simulink model "DSMC_params"  (R2020a)
settings: Solver=FixedStepAuto  StartTime=0.0  StopTime=30  FixedStep=Ts  MaxStep=0.015  RelTol=1e-3
PreLoadFcn:
  | if ~exist('sim_HIL')
  |     sim_HIL=false;
  | end
  | if ~exist('usefilter')
  |     usefilter=false;
  | end
InitFcn:
  | load motorModel.mat
  | load expsetup
model workspace (MAT data in the model file):
  C = [50; 1]
  DSMC_params_sdosession = sldodialogs.data.SessionData
  DSMC_params_sdosession.Version = '3.0'
  DSMC_params_sdosession.Data.ModelName = 'DSMC_params'
  DSMC_params_sdosession.Data.ToolType = 'ResponseOptimization'
  DSMC_params_sdosession.Data.GUIOptions.NoPromptClose = 0
  DSMC_params_sdosession.Data.Workspace.LocalWorkspace.DesignVars(1) = param.Continuous
  DSMC_params_sdosession.Data.Workspace.LocalWorkspace.DesignVars(1).Scale_ = [4; 1]
  DSMC_params_sdosession.Data.Workspace.LocalWorkspace.DesignVars(1).Size_ = [2 1]
  DSMC_params_sdosession.Data.Workspace.LocalWorkspace.DesignVars(1).Value_ = [50; 1]
  DSMC_params_sdosession.Data.Workspace.LocalWorkspace.DesignVars(1).pID = paramid.Variable
  DSMC_params_sdosession.Data.Workspace.LocalWorkspace.DesignVars(1).pID.Name = 'C'
  DSMC_params_sdosession.Data.Workspace.LocalWorkspace.DesignVars(2) = param.Continuous
  DSMC_params_sdosession.Data.Workspace.LocalWorkspace.DesignVars(2).Minimum_ = 1e-05
  DSMC_params_sdosession.Data.Workspace.LocalWorkspace.DesignVars(2).Maximum_ = 0.99999
  DSMC_params_sdosession.Data.Workspace.LocalWorkspace.DesignVars(2).Scale_ = 0.25
  DSMC_params_sdosession.Data.Workspace.LocalWorkspace.DesignVars(2).Size_ = [1 1]
  DSMC_params_sdosession.Data.Workspace.LocalWorkspace.DesignVars(2).Value_ = 0.1
  DSMC_params_sdosession.Data.Workspace.LocalWorkspace.DesignVars(2).pID = paramid.Variable
  DSMC_params_sdosession.Data.Workspace.LocalWorkspace.DesignVars(2).pID.Name = 'del'
  DSMC_params_sdosession.Data.Workspace.LocalWorkspace.DesignVars(3) = param.Continuous
  DSMC_params_sdosession.Data.Workspace.LocalWorkspace.DesignVars(3).Minimum_ = 1e-05
  DSMC_params_sdosession.Data.Workspace.LocalWorkspace.DesignVars(3).Maximum_ = 50
  DSMC_params_sdosession.Data.Workspace.LocalWorkspace.DesignVars(3).Scale_ = 0.001
  DSMC_params_sdosession.Data.Workspace.LocalWorkspace.DesignVars(3).Size_ = [1 1]
  DSMC_params_sdosession.Data.Workspace.LocalWorkspace.DesignVars(3).Value_ = 1
  DSMC_params_sdosession.Data.Workspace.LocalWorkspace.DesignVars(3).pID = paramid.Variable
  DSMC_params_sdosession.Data.Workspace.LocalWorkspace.DesignVars(3).pID.Name = 'eta'
  DSMC_params_sdosession.Data.Workspace.LocalWorkspace.DesignVars(4) = param.Continuous
  DSMC_params_sdosession.Data.Workspace.LocalWorkspace.DesignVars(4).Minimum_ = 1
  DSMC_params_sdosession.Data.Workspace.LocalWorkspace.DesignVars(4).Maximum_ = 100
  DSMC_params_sdosession.Data.Workspace.LocalWorkspace.DesignVars(4).Size_ = [1 1]
  DSMC_params_sdosession.Data.Workspace.LocalWorkspace.DesignVars(4).Value_ = 20
  DSMC_params_sdosession.Data.Workspace.LocalWorkspace.DesignVars(4).pID = paramid.Variable
  DSMC_params_sdosession.Data.Workspace.LocalWorkspace.DesignVars(4).pID.Name = 'gamm'
  DSMC_params_sdosession.Data.Workspace.LocalWorkspace.DesignVars(5) = param.Continuous
  DSMC_params_sdosession.Data.Workspace.LocalWorkspace.DesignVars(5).Minimum_ = 1e-05
  DSMC_params_sdosession.Data.Workspace.LocalWorkspace.DesignVars(5).Maximum_ = 0.99999
  DSMC_params_sdosession.Data.Workspace.LocalWorkspace.DesignVars(5).Scale_ = 0.5
  DSMC_params_sdosession.Data.Workspace.LocalWorkspace.DesignVars(5).Size_ = [1 1]
  DSMC_params_sdosession.Data.Workspace.LocalWorkspace.DesignVars(5).Value_ = 0.1
  DSMC_params_sdosession.Data.Workspace.LocalWorkspace.DesignVars(5).pID = paramid.Variable
  DSMC_params_sdosession.Data.Workspace.LocalWorkspace.DesignVars(5).pID.Name = 'qT'
  DSMC_params_sdosession.Data.Workspace.LocalWorkspace.DesignVars(6) = param.Continuous
  DSMC_params_sdosession.Data.Workspace.LocalWorkspace.DesignVars(6).Minimum_ = 1e-05
  DSMC_params_sdosession.Data.Workspace.LocalWorkspace.DesignVars(6).Maximum_ = 50
  DSMC_params_sdosession.Data.Workspace.LocalWorkspace.DesignVars(6).Scale_ = 0.5
  DSMC_params_sdosession.Data.Workspace.LocalWorkspace.DesignVars(6).Size_ = [1 1]
  DSMC_params_sdosession.Data.Workspace.LocalWorkspace.DesignVars(6).Value_ = 1
  DSMC_params_sdosession.Data.Workspace.LocalWorkspace.DesignVars(6).pID = paramid.Variable
  DSMC_params_sdosession.Data.Workspace.LocalWorkspace.DesignVars(6).pID.Name = 'vphi'
  DSMC_params_sdosession.Data.Workspace.LocalWorkspace.DesignVars(7) = param.Continuous
  DSMC_params_sdosession.Data.Workspace.LocalWorkspace.DesignVars(7).Minimum_ = 1e-05
  DSMC_params_sdosession.Data.Workspace.LocalWorkspace.DesignVars(7).Maximum_ = 50
  DSMC_params_sdosession.Data.Workspace.LocalWorkspace.DesignVars(7).Scale_ = 0.5
  DSMC_params_sdosession.Data.Workspace.LocalWorkspace.DesignVars(7).Size_ = [1 1]
  DSMC_params_sdosession.Data.Workspace.LocalWorkspace.DesignVars(7).Value_ = 10
  DSMC_params_sdosession.Data.Workspace.LocalWorkspace.DesignVars(7).pID = paramid.Variable
  DSMC_params_sdosession.Data.Workspace.LocalWorkspace.DesignVars(7).pID.Name = 'xiT'
  DSMC_params_sdosession.Data.Workspace.LocalWorkspace.posErr = Simulink.SimulationData.Signal
  DSMC_params_sdosession.Data.Workspace.LocalWorkspace.posErr.PortType = 'outport'
  DSMC_params_sdosession.Data.Workspace.LocalWorkspace.posErr.Version = 1
  DSMC_params_sdosession.Data.Workspace.LocalWorkspace.posErr.BlockPath = Simulink.SimulationData.BlockPath
  DSMC_params_sdosession.Data.Workspace.LocalWorkspace.posErr.BlockPath.path = {'DSMC_params/Visualization/Minus'}
  DSMC_params_sdosession.Data.Workspace.LocalWorkspace.posErrTracking = sdo.requirements.SignalTracking
  DSMC_params_sdosession.Data.Workspace.LocalWorkspace.posErrTracking.any.ReferenceSignal = timeseries
  DSMC_params_sdosession.Data.Workspace.LocalWorkspace.posErrTracking.any.ReferenceSignal.Name = 'unnamed'
  DSMC_params_sdosession.Data.Workspace.LocalWorkspace.posErrTracking.any.ReferenceSignal.DataInfo = tsdata.datametadata
  DSMC_params_sdosession.Data.Workspace.LocalWorkspace.posErrTracking.any.ReferenceSignal.DataInfo.Interpolation = tsdata.interpolation
  DSMC_params_sdosession.Data.Workspace.LocalWorkspace.posErrTracking.any.ReferenceSignal.DataInfo.Interpolation.Fhandle : function handle (value not decoded)
  DSMC_params_sdosession.Data.Workspace.LocalWorkspace.posErrTracking.any.ReferenceSignal.DataInfo.Interpolation.Name = 'linear'
  DSMC_params_sdosession.Data.Workspace.LocalWorkspace.posErrTracking.any.ReferenceSignal.TimeInfo = tsdata.timemetadata
  DSMC_params_sdosession.Data.Workspace.LocalWorkspace.posErrTracking.any.ReferenceSignal.TimeInfo.Length = 2
  DSMC_params_sdosession.Data.Workspace.LocalWorkspace.posErrTracking.any.ReferenceSignal.TimeInfo.DuplicateTimes = 0
  DSMC_params_sdosession.Data.Workspace.LocalWorkspace.posErrTracking.any.ReferenceSignal.TimeInfo.Time_ = [0; 30]
  DSMC_params_sdosession.Data.Workspace.LocalWorkspace.posErrTracking.any.ReferenceSignal.TimeInfo.Initialized = 1
  DSMC_params_sdosession.Data.Workspace.LocalWorkspace.posErrTracking.any.ReferenceSignal.QualityInfo = tsdata.qualmetadata
  DSMC_params_sdosession.Data.Workspace.LocalWorkspace.posErrTracking.any.ReferenceSignal.Data_ = [0; 0]
  DSMC_params_sdosession.Data.Workspace.LocalWorkspace.posErrTracking.any.Weights = [1; 1]
  DSMC_params_sdosession.Data.Workspace.LocalWorkspace.posErrTracking.any.Type = '=='
  DSMC_params_sdosession.Data.Workspace.LocalWorkspace.posErrTracking.any.Method = 'SSE'
  DSMC_params_sdosession.Data.Workspace.LocalWorkspace.posErrTracking.any.InterpolationTimes = 'Reference only'
  DSMC_params_sdosession.Data.Workspace.LocalWorkspace.posErrTracking.any.Normalize = 'on'
  DSMC_params_sdosession.Data.Workspace.LocalWorkspace.posErrTracking.any.RobustCost = 'on'
  DSMC_params_sdosession.Data.Workspace.LocalWorkspace.posErrTracking.any.RelTol = 0
  DSMC_params_sdosession.Data.Workspace.LocalWorkspace.posErrTracking.any.AbsTol = 0
  DSMC_params_sdosession.Data.Workspace.LocalWorkspace.posErrTracking.any.Name = ''
  DSMC_params_sdosession.Data.Workspace.LocalWorkspace.posErrTracking.any.Description = ''
  DSMC_params_sdosession.Data.Workspace.LocalWorkspace.posLowerBound = sdo.requirements.SignalBound
  DSMC_params_sdosession.Data.Workspace.LocalWorkspace.posLowerBound.sdo.requirements.Requirement.Data_ : srorequirement.piecewisedata (value not decoded)
  DSMC_params_sdosession.Data.Workspace.LocalWorkspace.posLowerBound.sdo.requirements.Requirement.Check_ = sdo.requirements.PiecewiseLinearCheck
  DSMC_params_sdosession.Data.Workspace.LocalWorkspace.posLowerBound.sdo.requirements.Requirement.Check_.Orientation = 'horizontal'
  DSMC_params_sdosession.Data.Workspace.LocalWorkspace.posLowerBound.sdo.requirements.Requirement.Check_.XScale = 'linear'
  DSMC_params_sdosession.Data.Workspace.LocalWorkspace.posUpperBound = sdo.requirements.SignalBound
  DSMC_params_sdosession.Data.Workspace.LocalWorkspace.posUpperBound.sdo.requirements.Requirement.Data_ : srorequirement.piecewisedata (value not decoded)
  DSMC_params_sdosession.Data.Workspace.LocalWorkspace.posUpperBound.sdo.requirements.Requirement.Check_ = sdo.requirements.PiecewiseLinearCheck
  DSMC_params_sdosession.Data.Workspace.LocalWorkspace.posUpperBound.sdo.requirements.Requirement.Check_.Orientation = 'horizontal'
  DSMC_params_sdosession.Data.Workspace.LocalWorkspace.posUpperBound.sdo.requirements.Requirement.Check_.XScale = 'linear'
  DSMC_params_sdosession.Data.Workspace.LocalWorkspace.velErr = Simulink.SimulationData.Signal
  DSMC_params_sdosession.Data.Workspace.LocalWorkspace.velErr.PortType = 'outport'
  DSMC_params_sdosession.Data.Workspace.LocalWorkspace.velErr.Version = 1
  DSMC_params_sdosession.Data.Workspace.LocalWorkspace.velErr.BlockPath = Simulink.SimulationData.BlockPath
  DSMC_params_sdosession.Data.Workspace.LocalWorkspace.velErr.BlockPath.path = {'DSMC_params/Visualization/Minus4'}
  DSMC_params_sdosession.Data.Workspace.HiddenWorkspace = []
  DSMC_params_sdosession.Data.ToolData.PlotManager.Plots.Class = 'sldoplots.TimePlot'
  DSMC_params_sdosession.Data.ToolData.PlotManager.Plots.Sources = {'posErr'}
  DSMC_params_sdosession.Data.ToolData.PlotManager.Tiling : java.lang.String (value not decoded)
  DSMC_params_sdosession.Data.ToolData.DialogManager = []
  DSMC_params_sdosession.Data.ToolData.ResponseOptimization.Options = sdo.OptimizeOptions
  DSMC_params_sdosession.Data.ToolData.ResponseOptimization.Options.OptimizedModel = 'SMC2'
  DSMC_params_sdosession.Data.ToolData.ResponseOptimization.Options.Version = 2
  DSMC_params_sdosession.Data.ToolData.ResponseOptimization.GUIOptions.ModelTimeOut = Inf
  DSMC_params_sdosession.Data.ToolData.ResponseOptimization.GUIOptions.ComputeOperatingPoint = 0
  DSMC_params_sdosession.Data.ToolData.ResponseOptimization.GUIOptions.ShowProgress = 1
  DSMC_params_sdosession.Data.ToolData.ResponseOptimization.GUIOptions.ShowParamTrajectory = 1
  DSMC_params_sdosession.Data.ToolData.ResponseOptimization.GUIOptions.UpdatePlots = 1
  DSMC_params_sdosession.Data.ToolData.ResponseOptimization.GUIOptions.UpdateModel = 1
  DSMC_params_sdosession.Data.ToolData.ResponseOptimization.GUIOptions.UpdateDesign = 'overwrite'
  DSMC_params_sdosession.Data.ToolData.ResponseOptimization.GUIOptions.SaveReport = 0
  DSMC_params_sdosession.Data.ToolData.ResponseOptimization.GUIOptions.SaveRequirementValue = 1
  DSMC_params_sdosession.Data.ToolData.ResponseOptimization.LinOptions = linearize.LinearizeOptions
  DSMC_params_sdosession.Data.ToolData.ResponseOptimization.RequirementOperatingPointSetup = []
  DSMC_params_sdosession.Data.ToolData.ResponseOptimization.LocalRequirements(1).Requirement = 'posErrTracking'
  DSMC_params_sdosession.Data.ToolData.ResponseOptimization.LocalRequirements(1).Source = {'posErr'}
  DSMC_params_sdosession.Data.ToolData.ResponseOptimization.LocalRequirements(1).Selected = 1
  DSMC_params_sdosession.Data.ToolData.ResponseOptimization.LocalRequirements(2).Requirement = 'posUpperBound'
  DSMC_params_sdosession.Data.ToolData.ResponseOptimization.LocalRequirements(2).Source = {'posErr'}
  DSMC_params_sdosession.Data.ToolData.ResponseOptimization.LocalRequirements(2).Selected = 1
  DSMC_params_sdosession.Data.ToolData.ResponseOptimization.LocalRequirements(3).Requirement = 'posLowerBound'
  DSMC_params_sdosession.Data.ToolData.ResponseOptimization.LocalRequirements(3).Source = {'posErr'}
  DSMC_params_sdosession.Data.ToolData.ResponseOptimization.LocalRequirements(3).Selected = 1
  DSMC_params_sdosession.Data.ToolData.ResponseOptimization.BlockRequirements = struct([])
  DSMC_params_sdosession.Data.ToolData.ResponseOptimization.LocalExperiments = struct([])
  DSMC_params_sdosession.Data.ToolData.ResponseOptimization.Cost.Type = 'SSE'
  DSMC_params_sdosession.Data.ToolData.ResponseOptimization.Cost.Robust = 'off'
  DSMC_params_sdosession.Data.ToolData.ResponseOptimization.DesignVariables = 'DesignVars'
  DSMC_params_sdosession.Data.ToolData.ResponseOptimization.UncertainVariables = ''
  DSMC_params_sdosession.Data.ToolData.ResponseOptimization.DataToPlot = 'posLowerBound'
  N = 10
  Ts_path = 0.015
  del = 0.1
  eta = 1
  gamm = 20
  nodeID = 4
  qT = 0.1
  vphi = 1
  xiT = 10
values from neighbouring files (symbols this model uses):
  Ts = 0.02    [PolynomialFit.m]
undefined symbols (not defined in the file or in its folder): k_lp, mModel, tau_lp, x28_000006_reduction
undefined symbols (not defined in the file): k, Xd
libraries: eeGeneralControl x1, dspsrcs4 x1, simulink_extras x1, simulink x1
settings Model: DataDictionary=MotorInfo.sldd  SimulationMode=accelerator  OrderedModelArguments=off  Creator=khoi  LastModifiedBy=khoi
settings OptimizationCC: DefaultParameterBehavior=Inlined  UseDivisionForNetSlopeComputation=on  GainParamInheritBuiltInType=on  UseFloatMulNetSlope=on  InlineInvariantSignals=on  EnhancedBackFolding=on  PassReuseOutputArgsAs=Individual arguments  ZeroExternalMemoryAtStartup=off  ZeroInternalMemoryAtStartup=off  EfficientFloat2IntCast=on  LifeSpan=50  SimCompilerOptimization=on  OptimizeBlockOrder=speed  DifferentSizesBufferReuse=on  OptimizationCustomize=off  EfficientTunableParamExpr=on
settings DebuggingCC: SignalInfNanChecking=warning  ParameterTunabilityLossMsg=error  AssertControl=DisableAll  SFUndirectedBroadcastEventsDiag=error
settings HardwareCC: ProdLongLongMode=on
settings ModelReferenceCC: EnableRefExpFcnMdlSchedulingChecks=off  EnableParallelModelReferenceBuilds=on  ModelReferenceMinAlgLoopOccurrences=on
settings SFSimCC: SimParseCustomCode=off  CompileTimeRecursionLimit=0  EnableRuntimeRecursion=off  MATLABDynamicMemAlloc=off
settings RTWCC: SystemTargetFile=ert.tlc  GenCodeOnly=on  TemplateMakefile=ert_default_tmf  GenerateReport=on  LaunchReport=on  CheckMdlBeforeBuild=Warning
settings CodeAppCC: ForceParamTrailComments=on  IgnoreCustomStorageClasses=off  OperatorAnnotations=on  SimulinkDataObjDesc=on  SFDataObjDesc=on  MATLABFcnDesc=on  InsertBlockDesc=on
settings ERTTargetCC: TargetLangStandard=C99 (ISO)  UtilityFuncGeneration=Shared location  GenerateSampleERTMain=on  SupportNonFinite=off  ParenthesesLevel=Maximum  CastingMode=Standards  GenerateSharedConstants=off  InlinedParameterPlacement=NonHierarchical  ERTCustomFileTemplate=example_file_process.tlc  EnableSignedLeftShifts=off  EnableSignedRightShifts=off

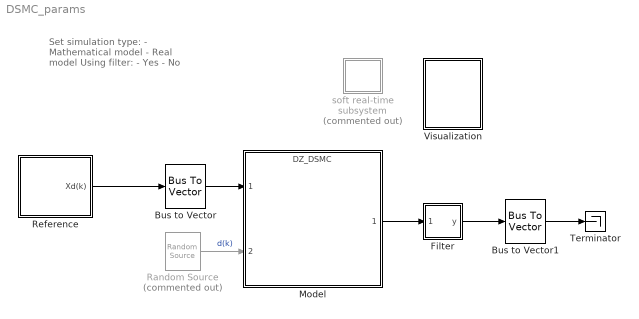
== system DSMC_params ==
  note: Set simulation type:
      | - Mathematical model
      | - Real model
      | Using filter:
      | - Yes
      | - No
  Bus to Vector : BusToVector
  Bus to Vector1 : BusToVector
  Filter : Subsystem
  Model : ModelReference  ModelNameDialog=DZ_DSMC.slx  ModelReferenceVersion=1.699  mask{Phi=mModel{nodeID,3}.A, Gam=mModel{nodeID,3}.B, nodeID=0, C=C, qT=qT, xiT=xiT, delt=del, vphi=vphi, eta=eta, gamm=gamm, Ts=Ts, N=N}
      mask prompts: Phi "State matrix"; Gam "Input matrix"; nodeID "Node ID"; C "Sliding vector"; qT "qT (0<1-qT<1)"; xiT "xiT >0"; delt "0<delta<1"; vphi "vphi>0"; eta "eta >0"; gamm "gamma (positive natural number)"; Ts "Sample tiem"; N "N order"
  Random Source : dspsrcs4/Random Source  Commented=on  SrcType=Gaussian  NormMethod=Ziggurat  CltLength=12  MinVal=0  MaxVal=1  MeanVal=0  VarVal=1  RepMode=Not repeatable  rawSeed=1  IsInherit=off  SampMode=Discrete  SampTime=Ts  SampFrame=1  DataType=Double  OutComplex=Real  OutputFrames=off
  Reference : Subsystem
  Terminator : Terminator
  Visualization : Subsystem
  soft real-time subsystem : Subsystem  Commented=on  mask{t_sample=0.01}
      mask prompts: t_sample "Sleep function interval (s)"
  wires:
  Reference/1(Xd(k)) -> Bus to Vector/1
  Filter/1(y) -> Bus to Vector1/1
  Random Source/1 -> Model/2  "d(k)"
  Bus to Vector/1 -> Model/1
  Bus to Vector1/1 -> Terminator/1
  Model/1 -> Filter/1(Input)

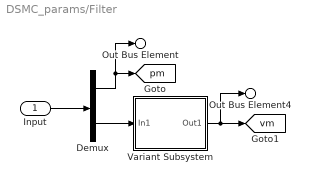
== system DSMC_params/Filter ==
  Input : Inport
  Demux : Demux  Outputs=2
  Variant Subsystem : Subsystem  Variant=on
  Out Bus Element4 : Outport  PortName=y  Element=dx
  Out Bus Element : Outport  PortName=y  Element=x
  tag scope: pm=global, vm=global
  wires:
  Demux/2 -> Variant Subsystem/1(In1)
  Demux/1 -> [pm], Out Bus Element/1
  Variant Subsystem/1(Out1) -> [vm], Out Bus Element4/1
  Input/1 -> Demux/1

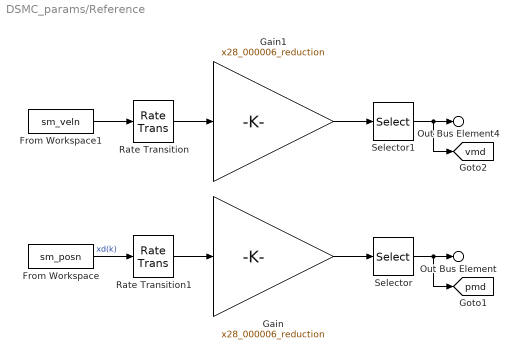
== system DSMC_params/Reference ==
  From Workspace : FromWorkspace  VariableName=sm_posn  SampleTime=Ts_path
  From Workspace1 : FromWorkspace  VariableName=sm_veln  SampleTime=Ts_path
  Gain : Gain  Gain=x28_000006_reduction
  Gain1 : Gain  Gain=x28_000006_reduction
  Rate Transition : RateTransition  OutPortSampleTime=Ts
  Rate Transition1 : RateTransition  OutPortSampleTime=Ts
  Selector : Selector  InputPortWidth=4  IndexOptions=Index vector (dialog)  Indices=nodeID  OutputSizes=1
  Selector1 : Selector  InputPortWidth=4  IndexOptions=Index vector (dialog)  Indices=nodeID  OutputSizes=1
  Out Bus Element : Outport  PortName=Xd(k)  Element=m.x
  Out Bus Element4 : Outport  PortName=Xd(k)  Element=m.dx
  tag scope: pmd=global, vmd=global
  wires:
  Selector1/1 -> [vmd], Out Bus Element4/1
  Selector/1 -> [pmd], Out Bus Element/1
  Gain/1 -> Selector/1
  From Workspace/1 -> Rate Transition1/1  "xd(k)"
  From Workspace1/1 -> Rate Transition/1
  Gain1/1 -> Selector1/1
  Rate Transition/1 -> Gain1/1
  Rate Transition1/1 -> Gain/1

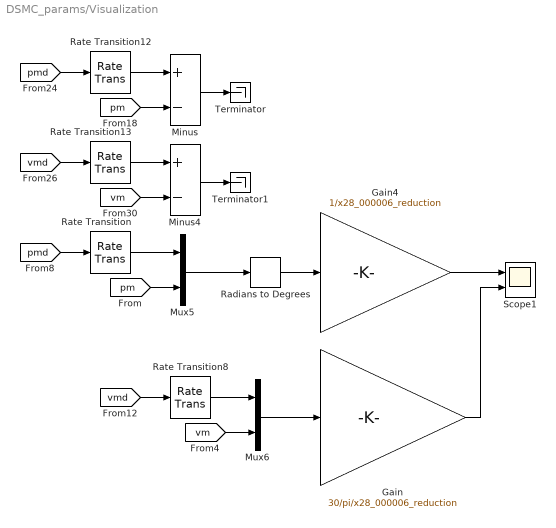
== system DSMC_params/Visualization ==
  Gain : Gain  Gain=30/pi/x28_000006_reduction
  Gain4 : Gain  Gain=1/x28_000006_reduction
  Minus : Sum  Inputs=+-
  Minus4 : Sum  Inputs=+-
  Mux5 : Mux  Inputs=2
  Mux6 : Mux  Inputs=2
  Radians to Degrees : simulink_extras/Transformations/Radians to Degrees
  Rate Transition{,8,12..13} (4 alike) : RateTransition
  Scope1 : Scope  NumInputPorts=2
  Terminator : Terminator
  Terminator1 : Terminator
  wires:
  Rate Transition8/1 -> Mux6/1
  Rate Transition13/1 -> Minus4/1
  Radians to Degrees/1 -> Gain4/1
  Rate Transition12/1 -> Minus/1
  [pm] -> Minus/2
  [vmd] -> Rate Transition13/1
  [vmd] -> Rate Transition8/1
  Gain4/1 -> Scope1/1
  Rate Transition/1 -> Mux5/1
  [vm] -> Minus4/2
  [pmd] -> Rate Transition12/1
  [vm] -> Mux6/2
  [pm] -> Mux5/2
  Mux5/1 -> Radians to Degrees/1
  [pmd] -> Rate Transition/1
  Minus/1 -> Terminator/1
  Mux6/1 -> Gain/1
  Gain/1 -> Scope1/2
  Minus4/1 -> Terminator1/1

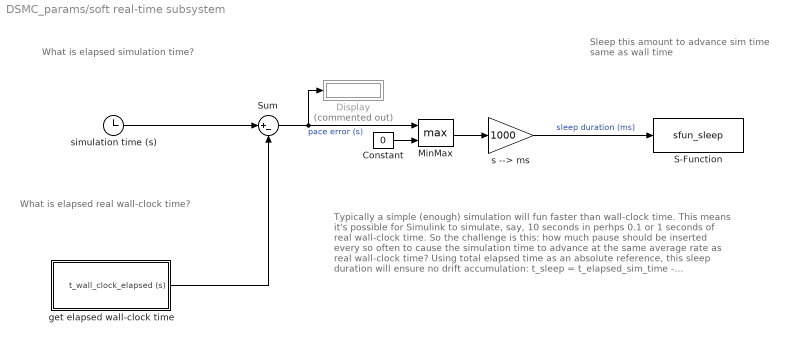
== system DSMC_params/soft real-time subsystem ==
  note: What is elapsed real
      | wall-clock time?
  note: What is elapsed
      | simulation time?
  note: Sleep this amount
      | to advance sim time
      | same as wall time
  note: Typically a simple (enough) simulation will fun faster than
      | wall-clock time. This means it's possible for Simulink to
      | simulate, say, 10 seconds in perhps 0.1 or 1 seconds of real
      | wall-clock time.
      |
      | So the challenge is this: how much pause should be inserted
      | every so often to cause the simulation time to advance at
      | the same average rate as real wall-clock time?
      |
      | Using total elapsed time as an absolute reference, this
      | sleep duration will ensure no drift accumulation:
      |
      | t_sleep = t_elapsed_sim_time - t_elapsed_wall_clock_time
      |
      | Pace error and Sleep() or usleep() resolution is system dependent
      | and likely around 10ms on Windows machines. Better on linux.
      |
      | Marc Compere
      | comperem@gmail.com
      | created : 28 May 2018
      | modified: 29 May 2018
      |
      | Reference:
      | Marc Compere (2022). S oft Real Time Block for Pacing Simulink Simulations (https://www.mathworks.com/matlabcentral/fileexchange/67520-soft-real-time-block-for-pacing-simulink-simulations), MATLAB Central File Exchange. Retrieved March 14, 2022.
  Constant : Constant  Value=0
  Display : Display  Commented=on
  MinMax : MinMax  Function=max  Inputs=2
  S-Function : S-Function  FunctionName=sfun_sleep  Parameters=t_sample  SFunctionDeploymentMode=off  EnableBusSupport=off
  Sum : Sum  Inputs=|+-
  get elapsed wall-clock time : Subsystem
  s --> ms : Gain  Gain=1000
  simulation time (s) : Clock
  wires:
  simulation time (s)/1 -> Sum/1
  Constant/1 -> MinMax/2
  get elapsed wall-clock time/1(t_wall_clock_elapsed (s)) -> Sum/2
  Sum/1 -> Display/1, MinMax/1  "pace error (s)"
  MinMax/1 -> s --> ms/1
  s --> ms/1 -> S-Function/1  "sleep duration (ms)"

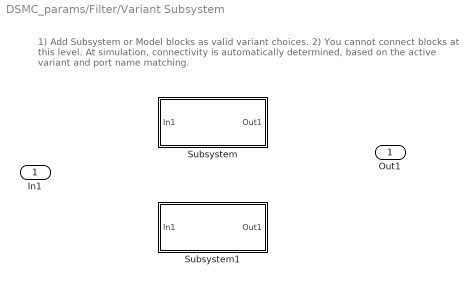
== system DSMC_params/Filter/Variant Subsystem ==
  note: 1) Add Subsystem or Model blocks as valid variant choices.
      | 2) You cannot connect blocks at this level. At simulation, connectivity is automatically
      | determined, based on the active variant and port name matching.
  In1 : Inport
  Subsystem : Subsystem  VariantControl=usefilter == true
  Subsystem1 : Subsystem  VariantControl=usefilter == false
  Out1 : Outport

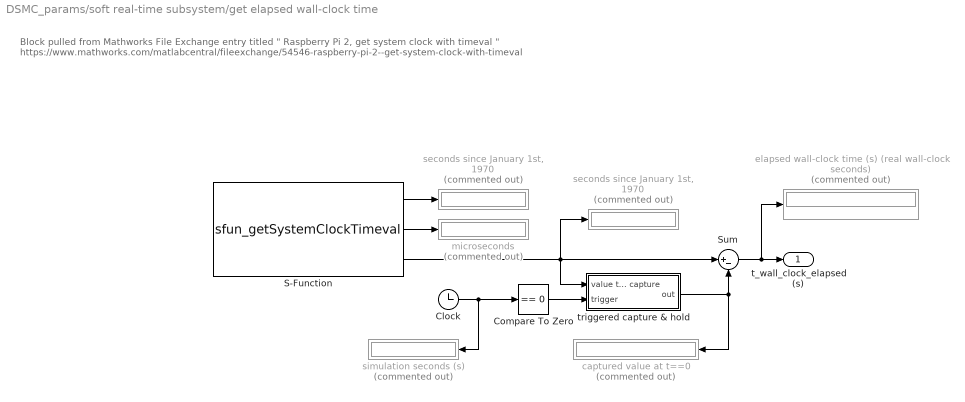
== system DSMC_params/soft real-time subsystem/get elapsed wall-clock time ==
  note: Block pulled from Mathworks File Exchange entry titled " Raspberry Pi 2, get system clock with timeval "
      |
      | https://www.mathworks.com/matlabcentral/fileexchange/54546-raspberry-pi-2--get-system-clock-with-timeval
  Clock : Clock
  Compare To Zero : simulink/Logic and Bit Operations/Compare To Zero  relop===  OutDataTypeStr=boolean
  S-Function : S-Function  FunctionName=sfun_getSystemClockTimeval  SFunctionDeploymentMode=off  EnableBusSupport=off
  Sum : Sum  Inputs=|+-
  captured value at t==0 : Display  Commented=on
  elapsed wall-clock time (s) (real wall-clock seconds) : Display  Commented=on
  microseconds : Display  Commented=on
  "seconds since January 1st, 1970" : Display  Commented=on
  "seconds since January 1st, 1970 " : Display  Commented=on
  simulation seconds (s) : Display  Commented=on
  triggered capture & hold : Subsystem
  t_wall_clock_elapsed (s) : Outport
  wires:
  triggered capture & hold/1(out) -> captured value at t==0/1, Sum/2
  S-Function/1 -> "seconds since January 1st, 1970 "/1
  Compare To Zero/1 -> triggered capture & hold/2(trigger)
  Sum/1 -> t_wall_clock_elapsed (s)/1, elapsed wall-clock time (s) (real wall-clock seconds)/1
  S-Function/2 -> microseconds/1
  S-Function/3 -> triggered capture & hold/1(value to capture), Sum/1, "seconds since January 1st, 1970"/1
  Clock/1 -> Compare To Zero/1, simulation seconds (s)/1

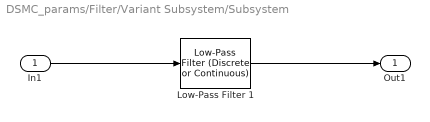
== system DSMC_params/Filter/Variant Subsystem/Subsystem ==
  In1 : Inport
  Low-Pass Filter 1 : eeGeneralControl/Low-Pass Filter (Discrete or Continuous)  K=k_lp(1)  T=tau_lp(1)  B=inf  A=-inf  init_option=Inherited from block input  x0=0  Ts=-1
  Out1 : Outport
  wires:
  In1/1 -> Low-Pass Filter 1/1
  Low-Pass Filter 1/1 -> Out1/1

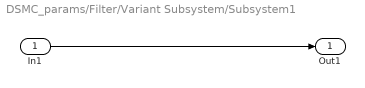
== system DSMC_params/Filter/Variant Subsystem/Subsystem1 ==
  In1 : Inport
  Out1 : Outport
  wires:
  In1/1 -> Out1/1

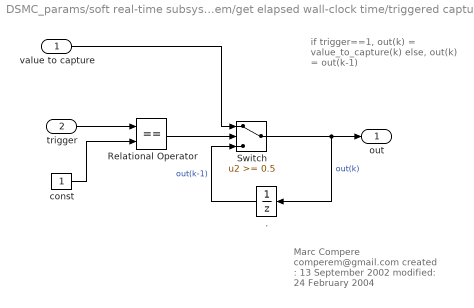
== system DSMC_params/soft real-time subsystem/get elapsed wall-clock time/triggered capture & hold ==
  note: Marc Compere
      | comperem@gmail.com
      | created  : 13 September 2002
      | modified: 24 February 2004
  note: if trigger==1,
      |    out(k) = value_to_capture(k)
      | else,
      |    out(k) = out(k-1)
  value to capture : Inport
  trigger : Inport  Port=2
  . : UnitDelay  SampleTime=-1  HasFrameUpgradeWarning=on
  Relational Operator : RelationalOperator  Operator===  RndMeth=Nearest
  Switch : Switch  Threshold=0.5  SaturateOnIntegerOverflow=on
  const : Constant
  out : Outport
  wires:
  trigger/1 -> Relational Operator/1
  const/1 -> Relational Operator/2
  Relational Operator/1 -> Switch/2
  Switch/1 -> ./1, out/1  "out(k)"
  value to capture/1 -> Switch/1
  ./1 -> Switch/3  "out(k-1)"
